simulink model "gpio_bidir"  (R2022a)
settings: Solver=VariableStepAuto  StartTime=0.0  StopTime=10.0  RelTol=1e-3
libraries: hdlBasic x6
settings Model: Creator=qwerty40  LastModifiedBy=bgodfrey
settings SolverCC: AlgebraicLoopSolver=TrustRegion
settings DataIOCC: ReturnWorkspaceOutputs=off
settings DebuggingCC: UnconnectedInputMsg=warning  UnconnectedOutputMsg=warning  UnconnectedLineMsg=warning  SFMachineParentedDataDiag=warning  ArithmeticOperatorsInVariantConditions=warning
settings SFSimCC: SimUseLocalCustomCode=off  CustomCodeUndefinedFunction=UseInterfaceOnly
settings RTWCC: RTWUseLocalCustomCode=off
settings CodeAppCC: StateflowObjectComments=on

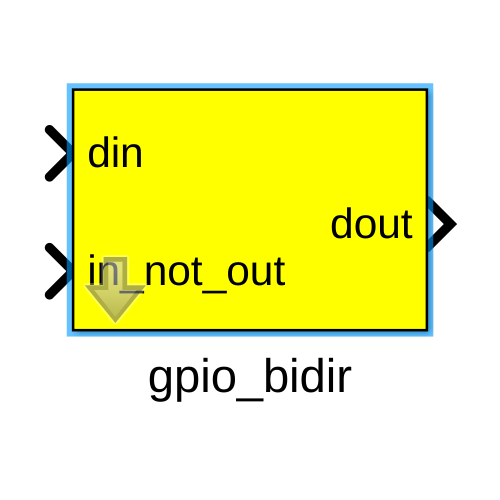
[thumbnail: Simulink's stored preview of the top-level diagram]
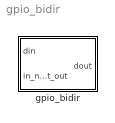
== system gpio_bidir ==
  gpio_bidir : Subsystem  Tag=xps:gpio_bidir  mask(gpio_bidir){io_group=gpio, bitwidth=4, bit_index=[0, 1, 2, 3]}
      mask prompts: io_group "I/O group"; bitwidth "Data bitwidth"; bit_index "GPIO bit index"
      mask help: Bi-directional GPIO interface.
      mask init:
      | gpio_bidir_mask;
      mask Help:
      | Inputs:
      | - din: data input (size set by Data bitwidth parameter in bits)
      | - in_not_out: The control signal, 1 for input and 0 for output.
      | 
      | Outputs:
      | - dout: The data output
      | 
      | When using bitwidths greater than one, you should specify a vector of bit indices to use. GPIO bit index should have the same number of elements as the I/O bitwidth.
      | 
      | See below for GPIO (GPIO bit indices correspond to TEST#):
      | 
      | Example: If you set Data bitwidth to 4, you might want you use GPIO bit indices [0, 1, 2, 3].
      | 
      | SNAP board
      | gpio:
      |     iostd: LVCMOS25
      |     loc:
      |       - B21 (TEST0)
      |       - C21 (TEST1)
      |       - B20 (TEST2)
      |       - A20 (TEST3)
      |       - H24 (TEST4)
      |       - H23 (TEST5)
      |       - B26 (TEST6)
      |       - R25 (TEST7)
      |       - L17 (TEST8)
      |       - K18 (TEST9)
      | led:
      |     iostd: LVCMOS25
      |     loc:
      |       - C13
      |       - C14
      |       - D13
      |       - D14
      |       - E12
      |       - E13
      mask TypeOptions io_group: led | gpio | sync_in | sync_out | zdok0 | zdok1

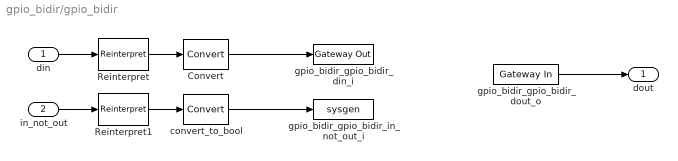
== system gpio_bidir/gpio_bidir ==
  din : Inport
  in_not_out : Inport  Port=2
  Convert : hdlBasic/Convert  gui_display_data_type=Fixed-point  arith_type=Unsigned  n_bits=4  bin_pt=0  float_type=Single  exp_bits=8  fraction_bits=24  quantization=Truncate  overflow=Wrap  en=off  latency=1  pipeline=off  XmcBlockStatus=1  maskContainerNames=group2  block_type=convert  block_config=sysgen:Convert_config  block_width=595  block_height=885
  Reinterpret : hdlBasic/Reinterpret  force_arith_type=on  arith_type=Unsigned  force_bin_pt=on  bin_pt=0  XmcBlockStatus=1  maskContainerNames=group1  block_type=reinterpret  block_config=sysgen:Reinterpret_config
  Reinterpret1 : hdlBasic/Reinterpret  force_arith_type=on  arith_type=Unsigned  force_bin_pt=on  bin_pt=0  XmcBlockStatus=1  maskContainerNames=group1  block_type=reinterpret  block_config=sysgen:Reinterpret_config
  convert_to_bool : hdlBasic/Convert  gui_display_data_type=Boolean  arith_type=Boolean  n_bits=16  bin_pt=14  float_type=Single  exp_bits=8  fraction_bits=24  quantization=Truncate  overflow=Wrap  en=off  latency=1  pipeline=off  XmcBlockStatus=1  maskContainerNames=group2  block_type=convert  block_config=sysgen:Convert_config  block_width=595  block_height=885
  gpio_bidir_gpio_bidir_din_i : hdlBasic/Gateway Out  inherit_from_input=off  hdl_port=on  rows=1  columns=1  UseAsDAC=off  DACChannel='1'  interface=None  automatic_assignment=on  address_offset=hex2dec('00')  intf_name=''  intf_description=''  timing_constraint=None  locs_specified=off  LOCs={}  io_standard={}  XmcBlockStatus=1  maskContainerNames=group4  block_type=gatewayout  block_config=sysgen:gateway_out_config  block_width_w=590  block_height_w=620  block_width=620  block_height=750
  gpio_bidir_gpio_bidir_dout_o : hdlBasic/Gateway In  gui_display_data_type=Fixed-point  arith_type=Unsigned  n_bits=4  bin_pt=0  preci_type=Single  exp_width=8  frac_width=24  rows=1  columns=1  quantization=Truncate  overflow=Wrap  period=1  UseAsADC=off  ADCChannel='1'  interface=None  automatic_assignment=on  address_offset=hex2dec('00')  intf_name=''  intf_description=''  default_value=0  timing_constraint=None  locs_specified=off  LOCs={}  io_standard={}  inherit_from_input=off  hdl_port=on  XmcBlockStatus=1  maskContainerNames=group4  block_type=gatewayin  block_config=sysgen:gateway_in_config  block_width_w=590  block_height_w=620  block_width=640  block_height=850
  gpio_bidir_gpio_bidir_in_not_out_i : S-Function  AncestorBlock=hdlBasic/Gateway Out  LoadFcn=obj = XmcLoadGUI(gcbh); obj.loadGUI();  FunctionName=sysgen  Parameters=ptable_  SFunctionDeploymentMode=off  EnableBusSupport=off  mask(Gateway Out Block){inherit_from_input=off, hdl_port=on, rows=1, columns=1, UseAsDAC=off, DACChannel='1', interface=None, automatic_assignment=on, address_offset=hex2dec('00'), intf_name='', intf_description='', timing_constraint=None, locs_specified=off, LOCs={}, io_standard={}, sginterface=, XmcBlockStatus=1, SD={'inherit_from_input'=>'Int','hdl_port'=>'Int','rows'=>'Int','columns'=>'Int','UseAsDAC'=>'Int','DACChannel'=>'String','interface'=>'Int','automatic_assignment'=>'Int','address_offset'=>'Int','intf_name'=>'String','intf_description'=>'String','timing_constraint'=>'Int','locs_specified'=>'Int','LOCs'=>'StringVector','io_standard'=>'StringVector','sginterface'=>'String','xinports'=>'DoubleVector','xoutports'=>'DoubleVector','block_type'=>'String'}, maskContainerNames=group4, block_type=gatewayout, block_config=sysgen:gateway_out_config, sg_icon_stat=60,20,1,1,white,yellow,1,cc31b7ac,right,,[ ],[ ], sg_mask_display=|, block_width_w=590, block_height_w=620, block_width=620, block_height=750}
      mask sg_mask_display=|
      | fprintf('','COMMENT: begin icon graphics');
      | patch([0 60 60 0 0 ],[0 0 20 20 0 ],[0.95 0.93 0.65 ]);
      | plot([0 60 60 0 0 ],[0 0 20 20 0 ]);
      | patch([25.55 28.44 30.44 32.44 34.44 30.44 27.55 25.55 ],[12.22 12.22 14.22 12.22 14.22 14.22 14.22 12.22 ],[1 1 1 ]);
      | patch([27.55 30.44 28.44 25.55 27.55 ],[10.22 10.22 12.22 12.22 10.22 ],[0.985 0.979 0.895 ]);
      | patch([25.55 28.44 30.44 27.55 25.55 ],[8.22 8.22 10.22 10.22 8.22 ],[1 1 1 ]);
      | patch([27.55 34.44 32.44 30.44 28.44 25.55 27.55 ],[6.22 6.22 8.22 6.22 8.22 8.22 6.22 ],[0.985 0.979 0.895 ]);
      | fprintf('','COMMENT: end icon graphics');
      | fprintf('','COMMENT: begin icon text');
      | color('black');port_label('input',1,' ');
      | color('black');port_label('output',1,'\fontsize{11pt}\bf Out ','texmode','on');
      | fprintf('','COMMENT: end icon text');
      mask prompts: inherit_from_input "Propagate data type to output"; hdl_port "Translate into output port"; rows "Number of rows"; columns "Number of columns"; UseAsDAC "Drive DAC Input"; DACChannel "DAC Channel ID"; automatic_assignment "Auto assign address offset"; address_offset "Address offset"; intf_name "Interface Name"; intf_description "Description"; timing_constraint "IOB timing constraint"; locs_specified "Specify IOB location constraints"; LOCs "IOB pad locations (cell array {'MSB', ..., 'LSB'})"; io_standard "IO Standards (specify as cell array {'MSB', ..., 'LSB'})"
      mask help:
      | Gateway out block. Converts Xilinx fixed-point or floating-point type inputs into outputs of type Simulink integer, single, double, or fixed-point.
      |
      | Hardware notes: In hardware, these blocks become top-level output ports or are discarded, depending on how they are configured.
      mask init:
      | obj = XmcInitGUI(gcbh, -1); ptable_ = obj.initGUI(); obj.setHorizontalOrientation();
      settings: OpenFcn=open_system(gcbh, 'mask');xmcPCSetDialogSize;
      mask Help: helpview(vmcHelp)
      mask Callback inherit_from_input: obj = XmcUpdateGUI(gcbh, @gatewayoutenablement, -1); obj.updateGUI()
      mask Callback hdl_port: obj = XmcUpdateGUI(gcbh, @gatewayoutenablement, -1); obj.updateGUI()
      mask Callback rows: obj = XmcUpdateGUI(gcbh, @gatewayoutenablement, -1); obj.updateGUI()
      mask Callback columns: obj = XmcUpdateGUI(gcbh, @gatewayoutenablement, -1); obj.updateGUI()
      mask Callback UseAsDAC: obj = XmcUpdateGUI(gcbh, @gatewayoutenablement, -1); obj.updateGUI()
      mask Callback DACChannel: obj = XmcUpdateGUI(gcbh, @gatewayoutenablement, -1); obj.updateGUI()
      mask TypeOptions interface: None | AXI4-Lite | Interrupt
      mask Callback interface: obj = XmcUpdateGUI(gcbh, @gatewayoutenablement, -1); obj.updateGUI()
      mask Callback automatic_assignment: obj = XmcUpdateGUI(gcbh, @gatewayoutenablement, -1); obj.updateGUI()
      mask Callback address_offset: obj = XmcUpdateGUI(gcbh, @gatewayoutenablement, -1); obj.updateGUI()
      mask Callback intf_name: obj = XmcUpdateGUI(gcbh, @gatewayoutenablement, -1); obj.updateGUI()
      mask Callback intf_description: obj = XmcUpdateGUI(gcbh, @gatewayoutenablement, -1); obj.updateGUI()
      mask TypeOptions timing_constraint: None | Data Rate | Data Rate;  Set 'FAST' Attribute
      mask Callback timing_constraint: obj = XmcUpdateGUI(gcbh, @gatewayoutenablement, -1); obj.updateGUI()
      mask Callback locs_specified: obj = XmcUpdateGUI(gcbh, @gatewayoutenablement, -1); obj.updateGUI()
      mask Callback LOCs: obj = XmcUpdateGUI(gcbh, @gatewayoutenablement, -1); obj.updateGUI()
      mask Callback io_standard: obj = XmcUpdateGUI(gcbh, @gatewayoutenablement, -1); obj.updateGUI()
      mask TypeOptions maskContainerNames: group4 | infoedit | tabcontainer1 | basictab | group1 | matrix_size | impltab | group2 | group3
      mask DialogControl DescGroupVar Prompt: Gateway Out
      mask DialogControl basictab Prompt: Basic
      mask DialogControl group1 Prompt: Output Type
      mask DialogControl matrix_size Prompt: Matrix size
      mask DialogControl impltab Prompt: Implementation
      mask DialogControl group2 Prompt: Interface Options
      mask DialogControl group3 Prompt: Constraints
      mask Display:
      | xmcDrawHDLBlockIcon();
      | fprintf('','COMMENT: begin icon text');
      | color('black');port_label('input',1,' ');
      | color('black');port_label('output',1,'\fontsize{11pt}\bf Out ','texmode','on');
      | fprintf('','COMMENT: end icon text');
  dout : Outport
  wires:
  in_not_out/1 -> Reinterpret1/1
  din/1 -> Reinterpret/1
  Reinterpret/1 -> Convert/1
  Reinterpret1/1 -> convert_to_bool/1
  Convert/1 -> gpio_bidir_gpio_bidir_din_i/1
  convert_to_bool/1 -> gpio_bidir_gpio_bidir_in_not_out_i/1
  gpio_bidir_gpio_bidir_dout_o/1 -> dout/1
